simulink model "Adaptive_Backstepping"  (R2020b)
settings: Solver=FixedStepAuto  StartTime=0.0  StopTime=500  FixedStep=1e-3  RelTol=1e-3
values from neighbouring files (symbols this model uses):
  g_par = 9.81    [init.m]
  J0 = 0.8*J_par    (= 154133333.333)    [init.m]
  J_par = (M_par*4*l_par^2)/12    (= 192666666.667)    [init.m]
  l_par = 34    [init.m]
  M0 = 0.5*M_par    (= 250000)    [init.m]
  M_par = 5e5    (= 500000)    [init.m]
  mu_x_par = 0.5*rho_par*cdx_par*Ax_par    (= 152.439)    [init.m]
  mu_y_par = 0.5*rho_par*cdy_par*Ay_par    (= 1.28880775561)    [init.m]
  muy0 = 0.1    [init.m]
  theta0 = deg2rad(15)    [init.m]
  x0 = 2    [init.m]
  y0 = -5    [init.m]
libraries: simulink x1
settings Model: Creator=chiara-s  LastModifiedBy=giorg

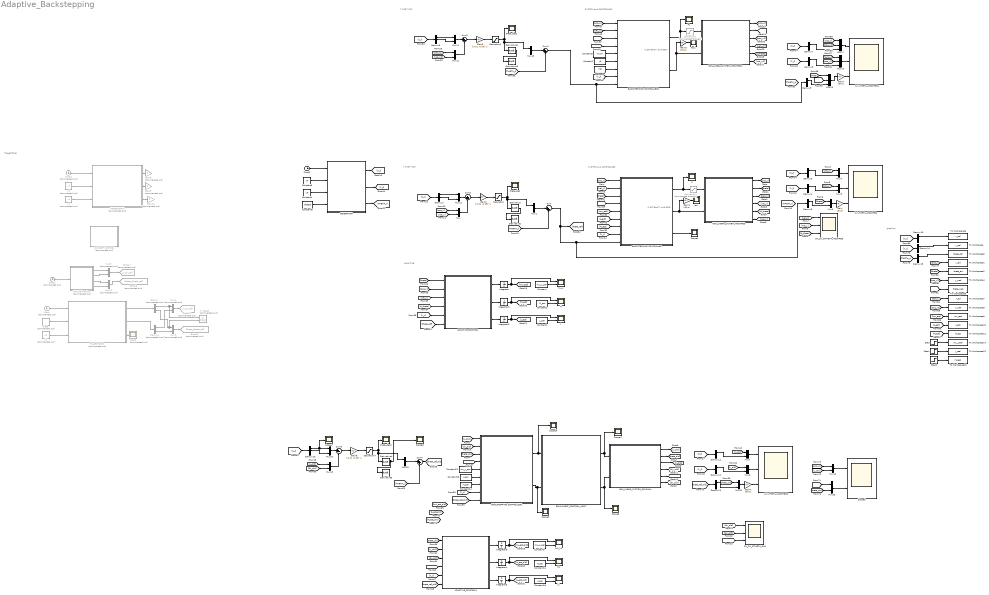
== system Adaptive_Backstepping ==
  note: graphics
  note: X outer loop
  note: ADAPTIVE
  note: SYSTEM and CONTROLLER
  note: TRAJECTORY
  note: -1.5075e-07 (s+0.995)
  note: SYSTEM and CONTROLLER
  note: X outer loop
  note: -1.5075e-07 (s+0.995)
  ADAPTIVE_CONTROL : MATLAB Function  TreatAsAtomicUnit=on
  ADAPTIVE_CONTROL1 : MATLAB Function  TreatAsAtomicUnit=on
  BACKSTEPPING CONTROLLER : Subsystem
  BACKSTEPPING CONTROLLER1 : Subsystem
  BACKSTEPPING CONTROLLER2 : Subsystem
  Clock : Clock  Commented=on
  Clock1 : Clock  Commented=on
  Clock2 : Clock  Commented=on
  Clock3 : Clock
  Constant : Constant  Value=mu_y_par
  Constant1 : Constant  Value=J_par
  Constant10 : Constant  Value=J_par
  Constant11 : Constant  Value=M_par
  Constant12 : Constant  Value=mu_y_par
  Constant13 : Constant  Value=J_par
  Constant14 : Constant  Value=M_par
  Constant2 : Constant  Value=M_par
  Constant3 : Constant  Value=muy0
  Constant4 : Constant  Value=y0
  Constant5 : Constant  Value=x0
  Constant6 : Constant  Value=theta0
  Constant7 : Constant  Value=J0
  Constant8 : Constant  Value=M0
  Constant9 : Constant  Value=mu_y_par
  DATASET NOSTRO1 : MATLAB Function  Commented=on  TreatAsAtomicUnit=on
  DX_DY_DTHETA_MODIFIED : Scope  NumInputPorts=3
  DX_DY_DTHETA_OLD : Scope  NumInputPorts=3
  Demux : Demux  Commented=on  Outputs=2
  Demux1 : Demux  Commented=on  Outputs=2
  Demux{2..16} (15 alike) : Demux  Outputs=3
  Derivative{,1..5} (6 alike) : Derivative
  EQUIVALENT_CONTROL_INPUT : MATLAB Function  TreatAsAtomicUnit=on
  F : Scope
  F1 : Scope
  GENERATOR : MATLAB Function  TreatAsAtomicUnit=on
  Gain{,1,3..4,7} (5 alike) : Gain  Gain=180/pi
  Gain10 : Gain  Commented=on
  Gain2 : Gain  Gain=[-0.01 -0.05]  Multiplication=Matrix(K*u)
  Gain5 : Gain  Gain=[-0.01 -0.05]  Multiplication=Matrix(K*u)
  Gain6 : Gain  Commented=on
  Gain8 : Gain  Gain=[-0.01 -0.05]  Multiplication=Matrix(K*u)
  Gain9 : Gain  Commented=on
  Goto12 : Goto  Commented=on  GotoTag=theta_dtheta_ref
  Goto13 : Goto  Commented=on  GotoTag=y_dy_ref
  Goto17 : Goto  Commented=on  GotoTag=y_dy_ref
  Goto18 : Goto  Commented=on  GotoTag=theta_dtheta_ref
  Integrator : Integrator  InitialCondition=muy0
  Integrator1 : Integrator  InitialCondition=M0
  Integrator2 : Integrator  InitialCondition=J0
  Integrator3 : Integrator  InitialCondition=muy0
  Integrator4 : Integrator  InitialCondition=M0
  Integrator5 : Integrator  InitialCondition=J0
  J : Scope  NumInputPorts=2
  J1 : Scope  NumInputPorts=2
  M : Scope  NumInputPorts=2
  M1 : Scope  NumInputPorts=2
  MATLAB Function : MATLAB Function  Commented=on  TreatAsAtomicUnit=on
  Mux{,4..8,11..12,14,18,20..23} (14 alike) : Mux  Inputs=2
  Mux{1,13,15..17,19} (6 alike) : Mux  Inputs=3
  Mux{2..3,9..10} (4 alike) : Mux  Commented=on  Inputs=2
  NON_LINEAR_SYSTEM_MODIFIED : Subsystem
  NON_LINEAR_SYSTEM_MODIFIED1 : Subsystem
  NON_LINEAR_SYSTEM_ORIGINAL : Subsystem
  Saturation : Saturate  UpperLimit=0.2  LowerLimit=-0.2
  Saturation1 : Saturate  UpperLimit=0.2  LowerLimit=-0.2
  Saturation2 : Saturate  Commented=through  UpperLimit=1e9  LowerLimit=0
  Saturation3 : Saturate  Commented=through  UpperLimit=1e9  LowerLimit=0
  Saturation4 : Saturate  UpperLimit=0.2  LowerLimit=-0.2
  Scope : Scope  Commented=on
  Scope{1..5,7..8} (7 alike) : Scope
  Scope6 : Scope  NumInputPorts=2
  Step : Step  Time=0  After=mu_y_par  SampleTime=0
  Step1 : Step  Time=0  After=J_par  SampleTime=0
  Step2 : Step  Time=0  After=M_par  SampleTime=0
  Sum : Sum  Inputs=|++
  Sum1 : Sum  Inputs=|++
  Sum2 : Sum  Inputs=|+-
  Sum3 : Sum  Inputs=|+-
  Sum4 : Sum  Inputs=|++
  Sum5 : Sum  Inputs=|+-
  TRAJECTORY2 : Subsystem  Commented=on
  TRAJECTORY3 : Subsystem  Commented=on
  To Workspace : ToWorkspace  VariableName=y_ref  SaveFormat=Timeseries  SampleTime=-1
  To Workspace1 : ToWorkspace  VariableName=y_ad  SaveFormat=Timeseries  SampleTime=-1
  To Workspace10 : ToWorkspace  VariableName=J_est  SaveFormat=Timeseries  SampleTime=-1
  To Workspace11 : ToWorkspace  VariableName=M_est  SaveFormat=Timeseries  SampleTime=-1
  To Workspace12 : ToWorkspace  VariableName=J_real  SaveFormat=Timeseries  SampleTime=-1
  To Workspace13 : ToWorkspace  VariableName=M_real  SaveFormat=Timeseries  SampleTime=-1
  To Workspace14 : ToWorkspace  VariableName=mu__real  SaveFormat=Timeseries  SampleTime=-1
  To Workspace2 : ToWorkspace  VariableName=theta_ad  SaveFormat=Timeseries  SampleTime=-1
  To Workspace3 : ToWorkspace  VariableName=theta_ref  SaveFormat=Timeseries  SampleTime=-1
  To Workspace4 : ToWorkspace  VariableName=y_nad  SaveFormat=Timeseries  SampleTime=-1
  To Workspace5 : ToWorkspace  VariableName=theta_nad  SaveFormat=Timeseries  SampleTime=-1
  To Workspace6 : ToWorkspace  VariableName=x_ref  SaveFormat=Timeseries  SampleTime=-1
  To Workspace7 : ToWorkspace  VariableName=x_ad  SaveFormat=Timeseries  SampleTime=-1
  To Workspace8 : ToWorkspace  VariableName=x_nad  SaveFormat=Timeseries  SampleTime=-1
  To Workspace9 : ToWorkspace  VariableName=mu_est  SaveFormat=Timeseries  SampleTime=-1
  XY Graph : simulink/Sinks/XY Graph  Commented=on  xmin=-5  xmax=30  ymin=-5  ymax=120  st=-1
  X_Y_THETA_MODIFIED : Scope  NumInputPorts=3
  X_Y_THETA_MODIFIED1 : Scope  NumInputPorts=3
  X_Y_THETA_MODIFIED2 : Scope  NumInputPorts=3
  mu_y : Scope  NumInputPorts=2
  mu_y1 : Scope  NumInputPorts=2
  tau : Scope
  tau1 : Scope
  theta : Constant  Commented=on  Value=theta0
  theta_des : Scope
  theta_des1 : Scope
  theta_des2 : Scope
  x1 : Constant  Commented=on  Value=x0
  y1 : Constant  Commented=on  Value=y0
  y2 : Constant  Commented=on  Value=y0
  wires:
  NON_LINEAR_SYSTEM_MODIFIED/1(pos_y) -> [pos_y]
  NON_LINEAR_SYSTEM_MODIFIED/2(theta) -> [theta]
  NON_LINEAR_SYSTEM_MODIFIED/3(pos_x) -> [pos_x]
  NON_LINEAR_SYSTEM_MODIFIED/4(vel_y) -> [vel_y]
  NON_LINEAR_SYSTEM_MODIFIED/5(d_theta) -> [d_theta]
  NON_LINEAR_SYSTEM_MODIFIED/6(vel_x) -> [vel_x]
  BACKSTEPPING CONTROLLER/1(F) -> Saturation3/1, F/1
  BACKSTEPPING CONTROLLER/2(tau) -> NON_LINEAR_SYSTEM_MODIFIED/2(tau), Gain1/1
  [vel_x] -> DX_DY_DTHETA_MODIFIED/1
  [vel_y] -> DX_DY_DTHETA_MODIFIED/2
  [d_theta] -> DX_DY_DTHETA_MODIFIED/3
  Gain1/1 -> tau/1
  Gain2/1 -> Saturation/1
  Mux11/1 -> Sum2/1
  Sum2/1 -> Gain2/1
  Saturation/1 -> theta_des/1, Mux1/1, Derivative/1
  Mux/1 -> Sum2/2
  [pos_x] -> Mux/1
  [vel_x] -> Mux/2
  NON_LINEAR_SYSTEM_ORIGINAL/3(pos_x) -> [x_old]
  NON_LINEAR_SYSTEM_ORIGINAL/1(pos_y) -> [y_old]
  NON_LINEAR_SYSTEM_ORIGINAL/4(vel_y) -> [dy_old]
  NON_LINEAR_SYSTEM_ORIGINAL/5(d_theta) -> [dtheta_old]
  NON_LINEAR_SYSTEM_ORIGINAL/2(theta) -> [theta_old]
  NON_LINEAR_SYSTEM_ORIGINAL/6(vel_x) -> [dx_old]
  EQUIVALENT_CONTROL_INPUT/1(T) -> NON_LINEAR_SYSTEM_ORIGINAL/1(T), Scope4/1
  EQUIVALENT_CONTROL_INPUT/2(phi) -> NON_LINEAR_SYSTEM_ORIGINAL/2(phi), Scope5/1
  [dx_old] -> DX_DY_DTHETA_OLD/1
  [dy_old] -> DX_DY_DTHETA_OLD/2
  [dtheta_old] -> DX_DY_DTHETA_OLD/3
  ADAPTIVE_CONTROL/3(J_est) -> Integrator2/1
  ADAPTIVE_CONTROL/2(M_est) -> Integrator1/1
  Constant/1 -> mu_y/2
  Constant2/1 -> M/2
  Constant1/1 -> J/2
  Demux/1 -> XY Graph/1, Mux2/1
  Demux1/1 -> Mux2/2
  Demux/2 -> XY Graph/2, Mux3/1
  Demux1/2 -> Mux3/2
  Mux5/1 -> X_Y_THETA_MODIFIED/2
  Mux4/1 -> X_Y_THETA_MODIFIED/1
  [pos_x] -> Mux4/1
  [pos_y] -> Mux5/1
  Clock/1 -> TRAJECTORY3/1(time)
  theta/1 -> TRAJECTORY3/2(theta0)
  y2/1 -> TRAJECTORY3/3(y0)
  TRAJECTORY3/1(z_des) -> Demux/1
  TRAJECTORY3/2(dz_des) -> Demux1/1
  TRAJECTORY3/3(ddz_des) -> Scope/1
  Mux2/1 -> Goto13/1
  Mux3/1 -> Goto12/1
  Mux6/1 -> Gain/1
  BACKSTEPPING CONTROLLER/3(qr_dot) -> Scope1/1
  [vel_y] -> BACKSTEPPING CONTROLLER/2(y_dot)
  [d_theta] -> BACKSTEPPING CONTROLLER/4(theta_dot)
  [theta] -> BACKSTEPPING CONTROLLER/3(theta)
  MATLAB Function/1(y) -> Mux9/1
  MATLAB Function/2(dy) -> Mux9/2
  MATLAB Function/3(theta) -> Mux10/1
  MATLAB Function/4(dtheta) -> Mux10/2
  Mux10/1 -> Goto18/1
  Mux9/1 -> Goto17/1
  Clock2/1 -> MATLAB Function/1(t)
  ADAPTIVE_CONTROL/1(muy_est) -> Integrator/1
  Integrator/1 -> mu_y/1, [mu_est]
  Integrator1/1 -> M/1, [M_est]
  Integrator2/1 -> J/1, [J_est]
  [mu_est] -> BACKSTEPPING CONTROLLER/5(mu_y)
  [M_est] -> BACKSTEPPING CONTROLLER/7(M)
  [J_est] -> BACKSTEPPING CONTROLLER/6(J)
  [pos_y] -> BACKSTEPPING CONTROLLER/1(y)
  [Y_r] -> BACKSTEPPING CONTROLLER/8(Y_r)
  [Y_r] -> ADAPTIVE_CONTROL/5(Y_r)
  [d_theta] -> ADAPTIVE_CONTROL/4(theta_dot)
  [vel_y] -> ADAPTIVE_CONTROL/3(y_dot)
  [pos_y] -> ADAPTIVE_CONTROL/2(y)
  [theta] -> ADAPTIVE_CONTROL/1(theta)
  Derivative/1 -> Derivative1/1
  [THETA_r] -> Sum/2
  [X_r] -> Demux2/1
  Demux2/1 -> Mux11/1
  Demux2/2 -> Mux11/2
  [X_r] -> Demux3/1
  Demux3/1 -> Mux4/2
  [Y_r] -> Demux4/1
  Demux4/1 -> Mux5/2
  Gain/1 -> X_Y_THETA_MODIFIED/3
  [theta] -> Mux6/1
  Demux5/1 -> Mux6/2
  [pos_y2] -> BACKSTEPPING CONTROLLER2/1(y)
  Constant3/1 -> BACKSTEPPING CONTROLLER2/5(mu_y)
  Constant7/1 -> BACKSTEPPING CONTROLLER2/6(J)
  [THETA_r] -> Sum1/2
  [theta2] -> BACKSTEPPING CONTROLLER2/3(theta)
  Demux6/2 -> Mux14/2
  Derivative2/1 -> Derivative3/1
  [X_r] -> Demux6/1
  Demux6/1 -> Mux14/1
  [vel_y2] -> BACKSTEPPING CONTROLLER2/2(y_dot)
  [Y_r] -> BACKSTEPPING CONTROLLER2/8(Y_r)
  [d_theta2] -> BACKSTEPPING CONTROLLER2/4(theta_dot)
  NON_LINEAR_SYSTEM_MODIFIED1/1(pos_y) -> [pos_y2]
  BACKSTEPPING CONTROLLER2/2(tau) -> NON_LINEAR_SYSTEM_MODIFIED1/2(tau), Gain3/1
  BACKSTEPPING CONTROLLER2/1(F) -> Saturation2/1, F1/1
  NON_LINEAR_SYSTEM_MODIFIED1/6(vel_x) -> [vel_x2]
  NON_LINEAR_SYSTEM_MODIFIED1/5(d_theta) -> [d_theta2]
  Gain5/1 -> Saturation1/1
  Gain3/1 -> tau1/1
  NON_LINEAR_SYSTEM_MODIFIED1/3(pos_x) -> [pos_x2]
  NON_LINEAR_SYSTEM_MODIFIED1/4(vel_y) -> [vel_y2]
  Mux12/1 -> Sum3/2
  [vel_x2] -> Mux12/2
  [pos_x2] -> Mux12/1
  Sum3/1 -> Gain5/1
  Saturation1/1 -> theta_des1/1, Mux13/1, Derivative2/1
  NON_LINEAR_SYSTEM_MODIFIED1/2(theta) -> [theta2]
  Constant8/1 -> BACKSTEPPING CONTROLLER2/7(M)
  Mux14/1 -> Sum3/1
  Gain7/1 -> X_Y_THETA_MODIFIED1/3
  [X_r] -> Demux7/1
  [Y_r] -> Demux8/1
  [theta2] -> Mux15/2
  Mux15/1 -> Gain7/1
  Demux9/1 -> Mux15/3
  [theta] -> Mux15/1
  Mux16/1 -> X_Y_THETA_MODIFIED1/2
  Mux17/1 -> X_Y_THETA_MODIFIED1/1
  [pos_x] -> Mux17/1
  [pos_x2] -> Mux17/2
  Demux7/1 -> Mux17/3
  Demux8/1 -> Mux16/3
  [pos_y2] -> Mux16/2
  [pos_y] -> Mux16/1
  Saturation2/1 -> NON_LINEAR_SYSTEM_MODIFIED1/1(F)
  Saturation3/1 -> NON_LINEAR_SYSTEM_MODIFIED/1(F)
  BACKSTEPPING CONTROLLER1/1(F) -> Scope3/1, EQUIVALENT_CONTROL_INPUT/1(F)
  BACKSTEPPING CONTROLLER1/2(tau) -> Scope2/1, EQUIVALENT_CONTROL_INPUT/2(tau)
  [y_old] -> BACKSTEPPING CONTROLLER1/1(y)
  [dy_old] -> BACKSTEPPING CONTROLLER1/2(y_dot)
  [theta_old] -> BACKSTEPPING CONTROLLER1/3(theta)
  [dtheta_old] -> BACKSTEPPING CONTROLLER1/4(theta_dot)
  [Y_r] -> BACKSTEPPING CONTROLLER1/8(Y_r)
  Sum5/1 -> Gain8/1
  Demux10/2 -> Mux20/2
  Derivative4/1 -> Scope8/1, Derivative5/1
  Demux10/1 -> Scope7/1, Mux20/1
  [THETA_r] -> Sum4/2
  [X_r] -> Demux10/1
  Mux19/1 -> Sum4/1
  [x_old] -> Mux18/1
  Mux18/1 -> Sum5/2
  Gain8/1 -> Saturation4/1
  Mux20/1 -> Sum5/1
  [dx_old] -> Mux18/2
  Saturation4/1 -> theta_des2/1, Mux19/1, Derivative4/1
  Sum4/1 -> [theta_ref_old]
  ADAPTIVE_CONTROL1/1(muy_est) -> Integrator3/1
  Integrator5/1 -> J1/1, [J_est_old]
  Integrator4/1 -> M1/1, [M_est_old]
  Constant11/1 -> M1/2
  ADAPTIVE_CONTROL1/3(J_est) -> Integrator5/1
  Constant10/1 -> J1/2
  Integrator3/1 -> mu_y1/1, [mu_est_old]
  Constant9/1 -> mu_y1/2
  ADAPTIVE_CONTROL1/2(M_est) -> Integrator4/1
  [dy_old] -> ADAPTIVE_CONTROL1/3(y_dot)
  [theta_old] -> ADAPTIVE_CONTROL1/1(theta)
  [y_old] -> ADAPTIVE_CONTROL1/2(y)
  [dtheta_old] -> ADAPTIVE_CONTROL1/4(theta_dot)
  [Y_r] -> ADAPTIVE_CONTROL1/5(Y_r)
  [theta_ref_old] -> ADAPTIVE_CONTROL1/6(THETA_r)
  Demux13/1 -> Mux21/2
  [Y_r] -> Demux12/1
  [X_r] -> Demux11/1
  Gain4/1 -> X_Y_THETA_MODIFIED2/3
  Mux21/1 -> Gain4/1
  Demux12/1 -> Mux8/2
  Mux7/1 -> X_Y_THETA_MODIFIED2/1
  Mux8/1 -> X_Y_THETA_MODIFIED2/2
  Demux11/1 -> Mux7/2
  [y_old] -> Mux8/1
  [theta_old] -> Mux21/1
  [x_old] -> Mux7/1
  [theta_ref_old] -> Demux13/1
  Constant12/1 -> BACKSTEPPING CONTROLLER1/5(mu_y)
  Constant13/1 -> BACKSTEPPING CONTROLLER1/6(J)
  Constant14/1 -> BACKSTEPPING CONTROLLER1/7(M)
  GENERATOR/3(THETA_r) -> [THETA_r]
  [y_old] -> Mux22/2
  [pos_y2] -> Mux22/1
  [theta2] -> Mux23/1
  [theta_old] -> Mux23/2
  Mux23/1 -> Scope6/2
  Mux22/1 -> Scope6/1
  Sum/1 -> [theta_ref], Demux5/1, BACKSTEPPING CONTROLLER/9(THETA_r)
  Sum1/1 -> Demux9/1, BACKSTEPPING CONTROLLER2/9(THETA_r)
  [theta_ref_old] -> BACKSTEPPING CONTROLLER1/9(THETA_r)
  [theta_ref] -> ADAPTIVE_CONTROL/6(THETA_r)
  TRAJECTORY2/1(x_ref) -> Gain6/1
  TRAJECTORY2/3(theta_ref) -> Gain10/1
  y1/1 -> TRAJECTORY2/3(y0)
  TRAJECTORY2/2(y_ref) -> Gain9/1
  x1/1 -> TRAJECTORY2/2(x0)
  Clock1/1 -> TRAJECTORY2/1(time)
  Constant4/1 -> GENERATOR/3(y0)
  Clock3/1 -> GENERATOR/1(time)
  Constant6/1 -> GENERATOR/4(theta0)
  Constant5/1 -> GENERATOR/2(x0)
  GENERATOR/1(X_r) -> [X_r]
  GENERATOR/2(Y_r) -> [Y_r]
  [Y_r] -> Demux14/1
  [THETA_r] -> Demux15/1
  [theta] -> To Workspace2/1
  [pos_y] -> To Workspace1/1
  Demux14/1 -> To Workspace/1
  Demux15/1 -> To Workspace3/1
  [theta2] -> To Workspace5/1
  [pos_y2] -> To Workspace4/1
  Demux16/1 -> To Workspace6/1
  [X_r] -> Demux16/1
  [pos_x] -> To Workspace7/1
  [pos_x2] -> To Workspace8/1
  Mux13/1 -> Sum1/1
  Mux1/1 -> Sum/1
  [mu_est] -> To Workspace9/1
  [J_est] -> To Workspace10/1
  [M_est] -> To Workspace11/1
  Step/1 -> To Workspace14/1
  Step1/1 -> To Workspace12/1
  Step2/1 -> To Workspace13/1

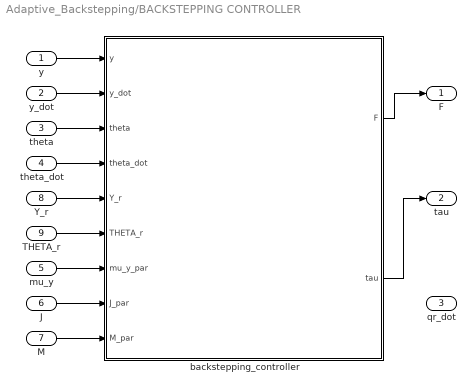
== system Adaptive_Backstepping/BACKSTEPPING CONTROLLER ==
  y : Inport
  y_dot : Inport  Port=2
  theta : Inport  Port=3
  theta_dot : Inport  Port=4
  mu_y : Inport  Port=5
  J : Inport  Port=6
  M : Inport  Port=7
  Y_r : Inport  Port=8
  THETA_r : Inport  Port=9
  backstepping_controller : MATLAB Function  TreatAsAtomicUnit=on
  F : Outport
  tau : Outport  Port=2
  qr_dot : Outport  Port=3
  wires:
  backstepping_controller/1(F) -> F/1
  backstepping_controller/2(tau) -> tau/1
  y/1 -> backstepping_controller/1(y)
  y_dot/1 -> backstepping_controller/2(y_dot)
  theta/1 -> backstepping_controller/3(theta)
  theta_dot/1 -> backstepping_controller/4(theta_dot)
  J/1 -> backstepping_controller/8(J_par)
  M/1 -> backstepping_controller/9(M_par)
  mu_y/1 -> backstepping_controller/7(mu_y_par)
  ? -> qr_dot/1
  Y_r/1 -> backstepping_controller/5(Y_r)
  THETA_r/1 -> backstepping_controller/6(THETA_r)

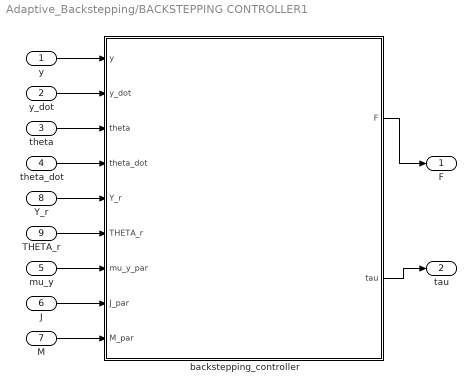
== system Adaptive_Backstepping/BACKSTEPPING CONTROLLER1 ==
  y : Inport
  y_dot : Inport  Port=2
  theta : Inport  Port=3
  theta_dot : Inport  Port=4
  mu_y : Inport  Port=5
  J : Inport  Port=6
  M : Inport  Port=7
  Y_r : Inport  Port=8
  THETA_r : Inport  Port=9
  backstepping_controller : MATLAB Function  TreatAsAtomicUnit=on
  F : Outport
  tau : Outport  Port=2
  wires:
  backstepping_controller/1(F) -> F/1
  backstepping_controller/2(tau) -> tau/1
  y/1 -> backstepping_controller/1(y)
  y_dot/1 -> backstepping_controller/2(y_dot)
  theta/1 -> backstepping_controller/3(theta)
  theta_dot/1 -> backstepping_controller/4(theta_dot)
  J/1 -> backstepping_controller/8(J_par)
  M/1 -> backstepping_controller/9(M_par)
  mu_y/1 -> backstepping_controller/7(mu_y_par)
  Y_r/1 -> backstepping_controller/5(Y_r)
  THETA_r/1 -> backstepping_controller/6(THETA_r)

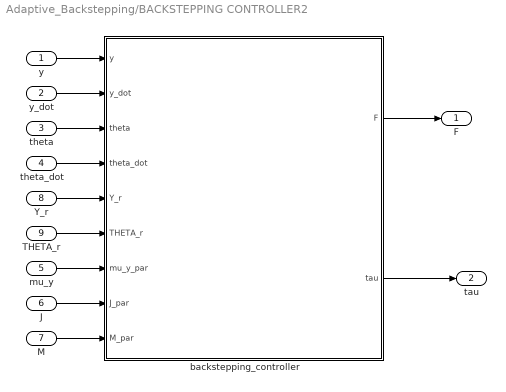
== system Adaptive_Backstepping/BACKSTEPPING CONTROLLER2 ==
  y : Inport
  y_dot : Inport  Port=2
  theta : Inport  Port=3
  theta_dot : Inport  Port=4
  mu_y : Inport  Port=5
  J : Inport  Port=6
  M : Inport  Port=7
  Y_r : Inport  Port=8
  THETA_r : Inport  Port=9
  backstepping_controller : MATLAB Function  TreatAsAtomicUnit=on
  F : Outport
  tau : Outport  Port=2
  wires:
  backstepping_controller/1(F) -> F/1
  backstepping_controller/2(tau) -> tau/1
  y/1 -> backstepping_controller/1(y)
  y_dot/1 -> backstepping_controller/2(y_dot)
  theta/1 -> backstepping_controller/3(theta)
  theta_dot/1 -> backstepping_controller/4(theta_dot)
  J/1 -> backstepping_controller/8(J_par)
  M/1 -> backstepping_controller/9(M_par)
  mu_y/1 -> backstepping_controller/7(mu_y_par)
  Y_r/1 -> backstepping_controller/5(Y_r)
  THETA_r/1 -> backstepping_controller/6(THETA_r)

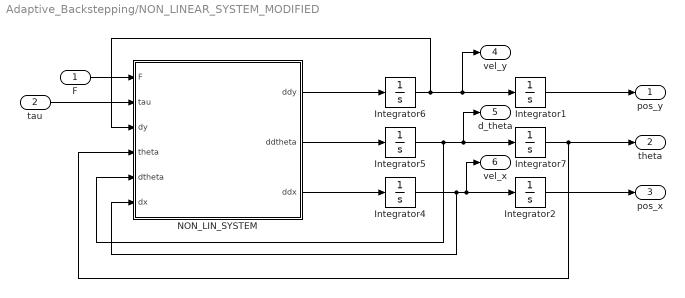
== system Adaptive_Backstepping/NON_LINEAR_SYSTEM_MODIFIED ==
  F : Inport
  tau : Inport  Port=2
  Integrator1 : Integrator  InitialCondition=y0
  Integrator2 : Integrator  InitialCondition=x0
  Integrator4 : Integrator
  Integrator5 : Integrator
  Integrator6 : Integrator
  Integrator7 : Integrator  InitialCondition=theta0
  NON_LIN_SYSTEM : MATLAB Function  TreatAsAtomicUnit=on
  pos_y : Outport
  theta : Outport  Port=2
  pos_x : Outport  Port=3
  vel_y : Outport  Port=4
  d_theta : Outport  Port=5
  vel_x : Outport  Port=6
  wires:
  Integrator2/1 -> pos_x/1
  Integrator7/1 -> NON_LIN_SYSTEM/4(theta), theta/1
  NON_LIN_SYSTEM/2(ddtheta) -> Integrator5/1
  tau/1 -> NON_LIN_SYSTEM/2(tau)
  Integrator1/1 -> pos_y/1
  F/1 -> NON_LIN_SYSTEM/1(F)
  Integrator6/1 -> Integrator1/1, vel_y/1, NON_LIN_SYSTEM/3(dy)
  Integrator4/1 -> NON_LIN_SYSTEM/6(dx), vel_x/1, Integrator2/1
  NON_LIN_SYSTEM/1(ddy) -> Integrator6/1
  Integrator5/1 -> NON_LIN_SYSTEM/5(dtheta), Integrator7/1, d_theta/1
  NON_LIN_SYSTEM/3(ddx) -> Integrator4/1

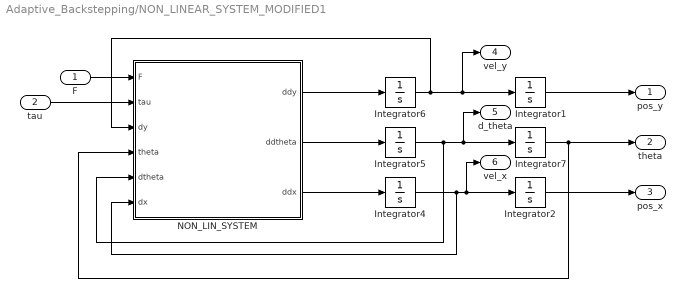
== system Adaptive_Backstepping/NON_LINEAR_SYSTEM_MODIFIED1 ==
  F : Inport
  tau : Inport  Port=2
  Integrator1 : Integrator  InitialCondition=y0
  Integrator2 : Integrator  InitialCondition=x0
  Integrator4 : Integrator
  Integrator5 : Integrator
  Integrator6 : Integrator
  Integrator7 : Integrator  InitialCondition=theta0
  NON_LIN_SYSTEM : MATLAB Function  TreatAsAtomicUnit=on
  pos_y : Outport
  theta : Outport  Port=2
  pos_x : Outport  Port=3
  vel_y : Outport  Port=4
  d_theta : Outport  Port=5
  vel_x : Outport  Port=6
  wires:
  Integrator2/1 -> pos_x/1
  Integrator7/1 -> NON_LIN_SYSTEM/4(theta), theta/1
  NON_LIN_SYSTEM/2(ddtheta) -> Integrator5/1
  tau/1 -> NON_LIN_SYSTEM/2(tau)
  Integrator1/1 -> pos_y/1
  F/1 -> NON_LIN_SYSTEM/1(F)
  Integrator6/1 -> Integrator1/1, vel_y/1, NON_LIN_SYSTEM/3(dy)
  Integrator4/1 -> NON_LIN_SYSTEM/6(dx), vel_x/1, Integrator2/1
  NON_LIN_SYSTEM/1(ddy) -> Integrator6/1
  Integrator5/1 -> NON_LIN_SYSTEM/5(dtheta), Integrator7/1, d_theta/1
  NON_LIN_SYSTEM/3(ddx) -> Integrator4/1

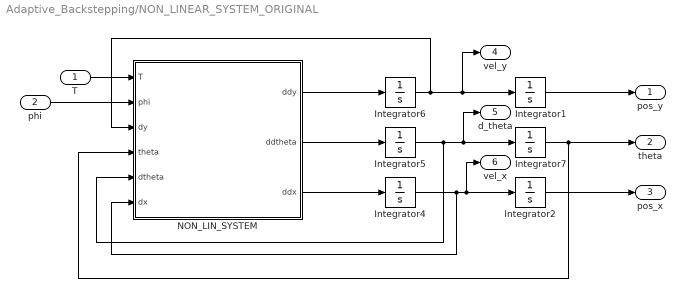
== system Adaptive_Backstepping/NON_LINEAR_SYSTEM_ORIGINAL ==
  T : Inport
  phi : Inport  Port=2
  Integrator1 : Integrator  InitialCondition=y0
  Integrator2 : Integrator  InitialCondition=x0
  Integrator4 : Integrator
  Integrator5 : Integrator
  Integrator6 : Integrator
  Integrator7 : Integrator  InitialCondition=theta0
  NON_LIN_SYSTEM : MATLAB Function  TreatAsAtomicUnit=on
  pos_y : Outport
  theta : Outport  Port=2
  pos_x : Outport  Port=3
  vel_y : Outport  Port=4
  d_theta : Outport  Port=5
  vel_x : Outport  Port=6
  wires:
  Integrator2/1 -> pos_x/1
  Integrator7/1 -> NON_LIN_SYSTEM/4(theta), theta/1
  NON_LIN_SYSTEM/2(ddtheta) -> Integrator5/1
  phi/1 -> NON_LIN_SYSTEM/2(phi)
  Integrator1/1 -> pos_y/1
  T/1 -> NON_LIN_SYSTEM/1(T)
  Integrator6/1 -> Integrator1/1, vel_y/1, NON_LIN_SYSTEM/3(dy)
  Integrator4/1 -> NON_LIN_SYSTEM/6(dx), vel_x/1, Integrator2/1
  NON_LIN_SYSTEM/1(ddy) -> Integrator6/1
  Integrator5/1 -> NON_LIN_SYSTEM/5(dtheta), Integrator7/1, d_theta/1
  NON_LIN_SYSTEM/3(ddx) -> Integrator4/1

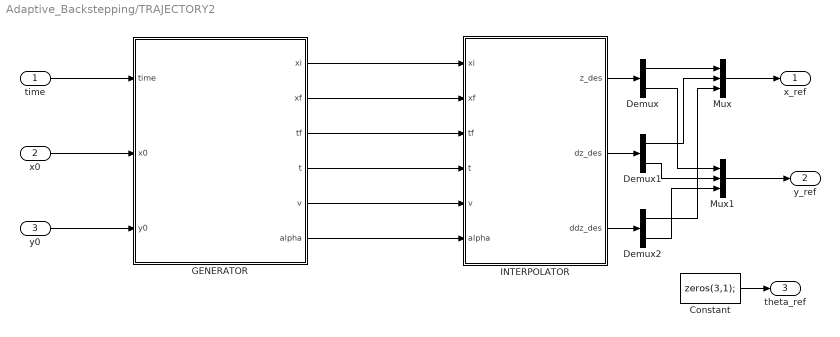
== system Adaptive_Backstepping/TRAJECTORY2 ==
  time : Inport
  x0 : Inport  Port=2
  y0 : Inport  Port=3
  Constant : Constant  Value=zeros(3,1);
  Demux : Demux  Outputs=2
  Demux1 : Demux  Outputs=2
  Demux2 : Demux  Outputs=2
  GENERATOR : MATLAB Function  TreatAsAtomicUnit=on
  INTERPOLATOR : MATLAB Function  TreatAsAtomicUnit=on
  Mux : Mux  Inputs=3
  Mux1 : Mux  Inputs=3
  x_ref : Outport
  y_ref : Outport  Port=2
  theta_ref : Outport  Port=3
  wires:
  GENERATOR/1(xi) -> INTERPOLATOR/1(xi)
  GENERATOR/2(xf) -> INTERPOLATOR/2(xf)
  GENERATOR/3(tf) -> INTERPOLATOR/3(tf)
  GENERATOR/4(t) -> INTERPOLATOR/4(t)
  GENERATOR/5(v) -> INTERPOLATOR/5(v)
  GENERATOR/6(alpha) -> INTERPOLATOR/6(alpha)
  time/1 -> GENERATOR/1(time)
  x0/1 -> GENERATOR/2(x0)
  y0/1 -> GENERATOR/3(y0)
  INTERPOLATOR/1(z_des) -> Demux/1
  INTERPOLATOR/2(dz_des) -> Demux1/1
  INTERPOLATOR/3(ddz_des) -> Demux2/1
  Constant/1 -> theta_ref/1
  Demux/1 -> Mux/1
  Demux1/1 -> Mux/2
  Demux2/1 -> Mux/3
  Mux/1 -> x_ref/1
  Mux1/1 -> y_ref/1
  Demux/2 -> Mux1/1
  Demux1/2 -> Mux1/2
  Demux2/2 -> Mux1/3

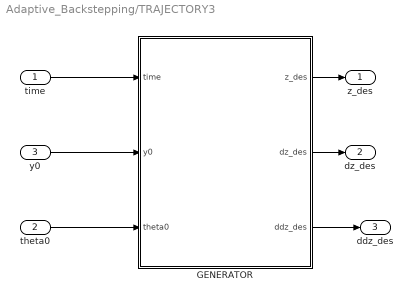
== system Adaptive_Backstepping/TRAJECTORY3 ==
  time : Inport
  theta0 : Inport  Port=2
  y0 : Inport  Port=3
  GENERATOR : MATLAB Function  TreatAsAtomicUnit=on
  z_des : Outport
  dz_des : Outport  Port=2
  ddz_des : Outport  Port=3
  wires:
  time/1 -> GENERATOR/1(time)
  GENERATOR/3(ddz_des) -> ddz_des/1
  GENERATOR/2(dz_des) -> dz_des/1
  GENERATOR/1(z_des) -> z_des/1
  theta0/1 -> GENERATOR/3(theta0)
  y0/1 -> GENERATOR/2(y0)

== matlab function Adaptive_Backstepping/ADAPTIVE_CONTROL ==
  data: theta input; y input; muy_est output; y_dot input; theta_dot input; Y_r input; THETA_r input; M_est output; J_est output; g_par parameter
function [muy_est, M_est, J_est] = fcn(theta, y, y_dot, theta_dot, Y_r, THETA_r, g_par)


R = zeros(3,3);
R = diag([10, 10^-4, 10^-8]);
u = zeros(3,1);

e_y = Y_r(1) - y;
e_y_dot = Y_r(2) - y_dot;
e_theta = THETA_r(1) - theta;
e_theta_dot = THETA_r(2) - theta_dot;

u(1) = inv(R(1,1))*y_dot*(e_y_dot+e_y);
u(2) = inv(R(2,2))*(e_y_dot+e_y)*(g_par+Y_r(3)+e_y_dot);
u(3) = inv(R(3,3))*(e_theta_dot+e_theta)*(THETA_r(3)+e_theta_dot);

muy_est = u(1);
M_est = u(2);
J_est = u(3);

end

== matlab function Adaptive_Backstepping/TRAJECTORY2/GENERATOR ==
  data: time input; xi output; xf output; tf output; t output; v output; alpha output; x0 input; y0 input
function  [xi, xf, tf, t, v, alpha] = fcn(time, x0, y0)

alpha = 0.1;

if time >= 0 && time < 50
    tf = 50;
    xi = [x0; y0];
    xf = [0; 0];
    t = time;
elseif time >= 50 && time < 150
    tf = 100;
    xi = [0; 0];
    xf = [0; 100];
    t = time - 50;
elseif time >= 150 && time < 250
    tf = 100;
    xi = [0; 100];
    xf = [20; 100];
    t = time - 150;
elseif time >= 250 && time < 350
    tf = 100; 
    xi = [20; 100];
    xf = [20; 0];
    t = time - 250;
elseif time >= 350 && time < 400
    tf = 50;
    xi = [20; 0];
    xf = xi;
    t = time - 350; 
else 
    tf = 1000;
    xi = [20; 0];
    xf = xi;
    t = time - 400; 
end
v = [(xf(1) - xi(1))/((1-alpha)*tf); (xf(2) - xi(2))/((1-alpha)*tf)];

end

== matlab function Adaptive_Backstepping/TRAJECTORY2/INTERPOLATOR ==
  data: xi input; z_des output; xf input; tf input; t input; v input; alpha input; dz_des output; ddz_des output
function [z_des, dz_des, ddz_des] = fcn(xi, xf, tf, t, v, alpha)

ta = alpha*tf; 
xa = (1/2)*v*ta;

if t >= 0 && t < ta
    ddz_des = v./ta;
    dz_des = ddz_des*t;
    z_des = xi + (1/2)*ddz_des*t^2;
elseif t >= ta && t < (tf-ta)
    ddz_des = [0; 0]; 
    dz_des = v; 
    z_des = xi + xa + dz_des*(t-ta);
elseif t >= (tf- ta) && t < tf
    ddz_des = -v./ta;
    dz_des = v + ddz_des*(t - (tf-ta));
    z_des = xi + xa + v*(tf-2*ta) + v*(t-(tf-ta)) + (1/2)*ddz_des*(t-(tf-ta))^2;
else 
    ddz_des = [0; 0];
    dz_des = [0; 0];
    z_des = xf;
end

end

== matlab function Adaptive_Backstepping/TRAJECTORY3/GENERATOR ==
  data: time input; y0 input; z_des output; dz_des output; ddz_des output; theta0 input
function  [z_des, dz_des, ddz_des] = fcn(time,y0,theta0)
t= time;
% pos_init = [x0;y0];
% z_des = pos_init + [20*sin(0.1*t); 10*sin(0.2*t)];
% dz_des = [cos(0.1*t)*2; cos(0.2*t)*2];
% ddz_des = [-sin(0.1*t)*0.2; -sin(0.2*t)*0.4];
pos_init = [y0;theta0];
z_des = pos_init + [20*sin(0.1*t); 10*pi/180*sin(0.2*t)];
dz_des = [cos(0.1*t)*2; pi/180*cos(0.2*t)*2];
ddz_des = [-sin(0.1*t)*0.2; -pi/180*sin(0.2*t)*0.4];
end

== matlab function Adaptive_Backstepping/MATLAB Function ==
  data: t input; y output; dy output; theta output; dtheta output; y0 parameter; theta0 parameter
function [y, dy, theta, dtheta] = fcn(t, y0, theta0)

y = y0 + t + t^2;
dy = 1 + 2*t;
theta = 0;
dtheta = 0;
end

== matlab function Adaptive_Backstepping/GENERATOR ==
  data: time input; x0 input; y0 input; X_r output; Y_r output; THETA_r output; theta0 input
function  [X_r, Y_r, THETA_r] = fcn(time, x0, y0, theta0)
t= time;
pos_init = [x0;y0];
z_des = pos_init + [20*sin(0.1*t); 10*sin(0.2*t)];
dz_des = [cos(0.1*t)*2; cos(0.2*t)*2];
ddz_des = [-sin(0.1*t)*0.2; -sin(0.2*t)*0.4];

X_r = [z_des(1); dz_des(1); ddz_des(1)];
Y_r = [z_des(2); dz_des(2); ddz_des(2)];
THETA_r = [0; 0; 0];
 
% X_r = [z_des(1); dz_des(1); ddz_des(1)];
% X_r = [0;0;0];
% Y_r = [z_des(2); dz_des(2); ddz_des(2)];
% THETA_r = [z_des(1); dz_des(1); ddz_des(1)];

% pos_init = [y0;theta0];
% z_des = pos_init + [20*sin(0.1*t); 10*pi/180*sin(0.2*t)];
% dz_des = [cos(0.1*t)*2; pi/180*cos(0.2*t)*2];
% ddz_des = [-sin(0.1*t)*0.2; -pi/180*sin(0.2*t)*0.4];
end

== matlab function Adaptive_Backstepping/BACKSTEPPING CONTROLLER2/backstepping_controller ==
  data: y input; F output; y_dot input; theta input; theta_dot input; Y_r input; THETA_r input; tau output; g_par parameter; mu_y_par input; J_par input; M_par input
function [F,tau] = fcn(y,y_dot,theta,theta_dot, Y_r, THETA_r,g_par, mu_y_par, J_par, M_par)
% v is pseudo control qdot_r
% Y_r and THETA_r are reference for position, velocity and acceleration

y_r = Y_r(1);
dy_r = Y_r(2);
ddy_r = Y_r(3);
theta_r = THETA_r(1);
dtheta_r = THETA_r(2);
ddtheta_r = THETA_r(3);

F = (M_par/cos(theta))*(ddy_r + 2*dy_r + y_r -y_dot*(2-mu_y_par/M_par) - y + g_par);
tau = J_par*(ddtheta_r + 2*dtheta_r + theta_r -2*theta_dot - theta);


% F = (M_par/cos(theta))*(Y_r(3) + 2*Y_r(2) + Y_r(1) -y_dot*(2-mu_y_par/M_par) - y + g_par);
% tau = J_par*(THETA_r(3) + 2*THETA_r(2) + THETA_r(1) -2*theta_dot - theta);

end

== matlab function Adaptive_Backstepping/DATASET NOSTRO1 ==
  data: T input; acc output; vel output; pos output
function [acc, vel, pos] = traj(T)

pos_init = single(zeros(3,1));
vel_init = single(zeros(3,1));
acc_init = single(zeros(3,1));
pos = pos_init;
vel = vel_init;
acc = acc_init;

c = 10;

if  T >= 0 && T < 50 %pausa iniziale
    pos = pos_init;
    vel = vel_init;
    acc = acc_init;

elseif T >= 50 && T < 300 %si muove su x e z
    tf = 250;
    pos_f = [75; 0; -20]*c;
    pos = single(pos_init + (pos_init - pos_f)*(15*((T-50)/tf)^4 - 6*((T-50)/tf)^5 - 10*((T-50)/tf)^3));
    vel = single((pos_init - pos_f)*(((60*(T-50)^3)/(tf^4)) - 30*(((T-50)^4)/(tf^5)) - 30*(((T-50)^2)/(tf^3))));
    acc = single((pos_init - pos_f)*(((180*(T-50)^2)/(tf^4)) - 120*(((T-50)^3)/(tf^5)) - 60*((T-50)/(tf^3))));
%     
%     rpy = [0; 0; 
elseif T >= 300 && T < 450 %si muove su y e z
    tf = 150;
    pos_init = [75; 0; -20]*c;
    pos_f = [75; -60; 0]*c;
    pos = single(pos_init + (pos_init - pos_f)*(15*((T-300)/tf)^4 - 6*((T-300)/tf)^5 - 10*((T-300)/tf)^3));
    vel = single((pos_init - pos_f)*(((60*(T-300)^3)/(tf^4)) - 30*(((T-300)^4)/(tf^5)) - 30*(((T-300)^2)/(tf^3))));
    acc = single((pos_init - pos_f)*(((180*(T-300)^2)/(tf^4)) - 120*(((T-300)^3)/(tf^5)) - 60*((T-300)/(tf^3))));
elseif T >= 450 && T < 750 % si muove su x e y e z
    tf = 300;
    pos_f = [10; 10; -30]*c;
    pos_init = [75; -60; 0]*c;
    pos = single(pos_init + (pos_init - pos_f)*(15*((T-450)/tf)^4 - 6*((T-450)/tf)^5 - 10*((T-450)/tf)^3));
    vel = single((pos_init - pos_f)*(((60*(T-450)^3)/(tf^4)) - 30*(((T-450)^4)/(tf^5)) - 30*(((T-450)^2)/(tf^3))));
    acc = single((pos_init - pos_f)*(((180*(T-450)^2)/(tf^4)) - 120*(((T-450)^3)/(tf^5)) - 60*((T-450)/(tf^3))));
elseif T >= 750 && T < 1000
    tf = 250;
    pos_init = [10; 10; -30]*c;
    pos_f = [0; 0; 0]*c;
    pos = single(pos_init + (pos_init - pos_f)*(15*((T-750)/tf)^4 - 6*((T-750)/tf)^5 - 10*((T-750)/tf)^3));
    vel = single((pos_init - pos_f)*(((60*(T-750)^3)/(tf^4)) - 30*(((T-750)^4)/(tf^5)) - 30*(((T-750)^2)/(tf^3))));
    acc = single((pos_init - pos_f)*(((180*(T-750)^2)/(tf^4)) - 120*(((T-750)^3)/(tf^5)) - 60*((T-750)/(tf^3))));
else
    pos_init = [0; 0; 0];
    pos = single(pos_init);
    vel = single(zeros(3,1));
    acc = single(zeros(3,1));
end 
end

== matlab function Adaptive_Backstepping/BACKSTEPPING CONTROLLER/backstepping_controller ==
  data: y input; F output; y_dot input; theta input; theta_dot input; Y_r input; THETA_r input; tau output; g_par parameter; mu_y_par input; J_par input; M_par input
function [F,tau] = fcn(y,y_dot,theta,theta_dot, Y_r, THETA_r,g_par, mu_y_par, J_par, M_par)
% v is pseudo control qdot_r
% Y_r and THETA_r are reference for position, velocity and acceleration
% F = M_par*(-2*y_dot - y + g_par + (mu_y_par/M_par)*y_dot)/cos(theta);
% tau = -J_par*(theta + 2*theta_dot);
y_r = Y_r(1);
dy_r = Y_r(2);
ddy_r = Y_r(3);
theta_r = THETA_r(1);
dtheta_r = THETA_r(2);
ddtheta_r = THETA_r(3);

F = (M_par/cos(theta))*(ddy_r + 2*dy_r + y_r -y_dot*(2-mu_y_par/M_par) - y + g_par);
tau = J_par*(ddtheta_r + 2*dtheta_r + theta_r -2*theta_dot - theta);

end

== matlab function Adaptive_Backstepping/NON_LINEAR_SYSTEM_MODIFIED1/NON_LIN_SYSTEM ==
  data: F input; ddy output; tau input; dy input; theta input; dtheta input; dx input; ddtheta output; ddx output; M_par parameter; mu_x_par parameter; J_par parameter; l_par parameter; mu_y_par parameter; g_par parameter
function [ddy, ddtheta, ddx] = fcn(F, tau, dy, theta, dtheta, dx, M_par, mu_x_par, J_par, l_par, mu_y_par, g_par)

% u = [F,tau] here we consider alligned thrusther with y axis and torque
% tau 
ddx = M_par^-1*(-F*sin(theta) - mu_x_par*dx);
ddtheta = J_par^-1*tau;
ddy = M_par^-1*(F*cos(theta) - mu_y_par*dy - M_par*g_par);


end

== matlab function Adaptive_Backstepping/ADAPTIVE_CONTROL1 ==
  data: theta input; y input; muy_est output; y_dot input; theta_dot input; Y_r input; THETA_r input; M_est output; J_est output; g_par parameter
function [muy_est, M_est, J_est] = fcn(theta, y, y_dot, theta_dot, Y_r, THETA_r, g_par)


R = zeros(3,3);
R = diag([10, 10^-4, 10^-8]);
u = zeros(3,1);

e_y = Y_r(1) - y;
e_y_dot = Y_r(2) - y_dot;
e_theta = THETA_r(1) - theta;
e_theta_dot = THETA_r(2) - theta_dot;

u(1) = inv(R(1,1))*y_dot*(e_y_dot+e_y);
u(2) = inv(R(2,2))*(e_y_dot+e_y)*(g_par+Y_r(3)+e_y_dot);
u(3) = inv(R(3,3))*(e_theta_dot+e_theta)*(THETA_r(3)+e_theta_dot);

muy_est = u(1);
M_est = u(2);
J_est = u(3);

end

== matlab function Adaptive_Backstepping/NON_LINEAR_SYSTEM_MODIFIED/NON_LIN_SYSTEM ==
  data: F input; ddy output; tau input; dy input; theta input; dtheta input; dx input; ddtheta output; ddx output; M_par parameter; mu_x_par parameter; J_par parameter; l_par parameter; mu_y_par parameter; g_par parameter
function [ddy, ddtheta, ddx] = fcn(F, tau, dy, theta, dtheta, dx, M_par, mu_x_par, J_par, l_par, mu_y_par, g_par)

% u = [F,tau] here we consider alligned thrusther with y axis and torque
% tau 
ddx = M_par^-1*(-F*sin(theta) - mu_x_par*dx);
ddtheta = J_par^-1*tau;
ddy = M_par^-1*(F*cos(theta) - mu_y_par*dy - M_par*g_par);


end

== matlab function Adaptive_Backstepping/NON_LINEAR_SYSTEM_ORIGINAL/NON_LIN_SYSTEM ==
  data: T input; ddy output; phi input; dy input; theta input; dtheta input; dx input; ddtheta output; ddx output; M_par parameter; mu_x_par parameter; J_par parameter; l_par parameter; mu_y_par parameter; g_par parameter
function [ddy, ddtheta, ddx] = fcn(T, phi, dy, theta, dtheta, dx, M_par, mu_x_par, J_par, l_par, mu_y_par, g_par)

ddx = M_par^-1*(-T*sin(theta+phi) - mu_x_par*dx);
ddtheta = J_par^-1*(-T*l_par*sin(phi));
ddy = M_par^-1*(T*cos(theta+phi) - mu_y_par*dy - M_par*g_par);


end

== matlab function Adaptive_Backstepping/BACKSTEPPING CONTROLLER1/backstepping_controller ==
  data: y input; F output; y_dot input; theta input; theta_dot input; Y_r input; THETA_r input; tau output; g_par parameter; mu_y_par input; J_par input; M_par input
function [F,tau] = fcn(y,y_dot,theta,theta_dot, Y_r, THETA_r,g_par, mu_y_par, J_par, M_par)
% v is pseudo control qdot_r
% Y_r and THETA_r are reference for position, velocity and acceleration
% F = M_par*(-2*y_dot - y + g_par + (mu_y_par/M_par)*y_dot)/cos(theta);
% tau = -J_par*(theta + 2*theta_dot);
y_r = Y_r(1);
dy_r = Y_r(2);
ddy_r = Y_r(3);
theta_r = THETA_r(1);
dtheta_r = THETA_r(2);
ddtheta_r = THETA_r(3);

F = (M_par/cos(theta))*(ddy_r + 2*dy_r + y_r -y_dot*(2-mu_y_par/M_par) - y + g_par);
tau = J_par*(ddtheta_r + 2*dtheta_r + theta_r -2*theta_dot - theta);

end

== matlab function Adaptive_Backstepping/EQUIVALENT_CONTROL_INPUT ==
  data: F input; T output; tau input; phi output; l_par parameter
function [T, phi] = fcn(F,tau, l_par)

phi = -atan2(tau,F*l_par);
T = F/cos(phi);



end
